simulink model "attitudeEstimation"  (R2018a)
settings: Solver=FixedStepAuto  StartTime=0.0  StopTime=10.0  RelTol=1e-3
undefined symbols (not defined in the file): SkywalkerX8
libraries: sharedTrackingLibrary x1
settings Model: Creator=David  LastModifiedBy=David

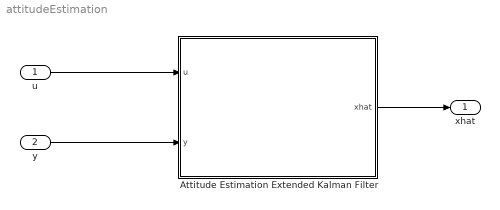
== system attitudeEstimation ==
  u : Inport  PortDimensions=4  SampleTime=SkywalkerX8.Sensors.EKF.Attitude.StateTransitionSampleTime
  y : Inport  Port=2  PortDimensions=3  SampleTime=SkywalkerX8.Sensors.EKF.Attitude.MeasurementSampleTime
  Attitude Estimation Extended Kalman Filter : Subsystem
      mask Display:
      | port_label('input', 1, '{\bf u} = [p, q, r, V_a]', 'texMode', 'On')
      | port_label('input', 2, '{\bf y} = [a_x, a_y, a_z]', 'texMode', 'On')
      | 
      | port_label('output', 1, '{\bf x_{est}} = [\Phi, \theta]', 'texMode', 'On')
  xhat : Outport
  wires:
  u/1 -> Attitude Estimation Extended Kalman Filter/1(u)
  y/1 -> Attitude Estimation Extended Kalman Filter/2(y)
  Attitude Estimation Extended Kalman Filter/1(xhat) -> xhat/1

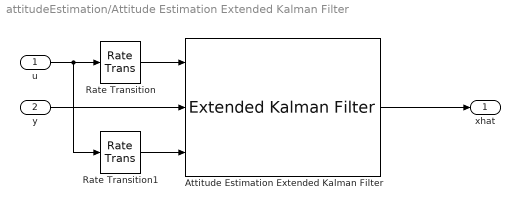
== system attitudeEstimation/Attitude Estimation Extended Kalman Filter ==
  u : Inport
  y : Inport  Port=2
  Attitude Estimation Extended Kalman Filter : sharedTrackingLibrary/Extended Kalman Filter  StateTransitionFcn=attitudeTransitionEstimate  HasStateTransitionJacobianFcn=on  StateTransitionJacobianFcn=attitudeTransitionEstimate_Jacobian  HasAdditiveProcessNoise=Additive  ProcessNoise=SkywalkerX8.Sensors.EKF.Attitude.ProcessCovarianceMatrix  HasTimeVaryingProcessNoise=off  HasStateTransitionFcnExtraArgument=1  InitialState=SkywalkerX8.Sensors.EKF.Attitude.InitialState  InitialStateCovariance=SkywalkerX8.Sensors.EKF.Attitude.InitialStateCovarianceMatrix  MeasurementFcn1=accelerometerMeasurementEstimate  HasMeasurementJacobianFcn1=on  MeasurementJacobianFcn1=accelerometerMeasurementEstimate_Jacobian  HasMeasurementEnablePort1=off  HasAdditiveMeasurementNoise1=Additive  MeasurementNoise1=SkywalkerX8.Sensors.EKF.Attitude.MeasurementCovarianceMatrix  HasTimeVaryingMeasurementNoise1=off  HasMeasurementFcnExtraArgument1=1  MeasurementFcn2=myMeasurementFcn  HasMeasurementJacobianFcn2=off  HasMeasurementEnablePort2=off  HasAdditiveMeasurementNoise2=Additive  MeasurementNoise2=1  HasTimeVaryingMeasurementNoise2=off  HasMeasurementFcnExtraArgument2=0  MeasurementFcn3=myMeasurementFcn  HasMeasurementJacobianFcn3=off  HasMeasurementEnablePort3=off  HasAdditiveMeasurementNoise3=Additive  MeasurementNoise3=1  HasTimeVaryingMeasurementNoise3=off  HasMeasurementFcnExtraArgument3=0  MeasurementFcn4=myMeasurementFcn  HasMeasurementJacobianFcn4=off  HasMeasurementEnablePort4=off  HasAdditiveMeasurementNoise4=Additive  MeasurementNoise4=1  HasTimeVaryingMeasurementNoise4=off  HasMeasurementFcnExtraArgument4=0  MeasurementFcn5=myMeasurementFcn  HasMeasurementJacobianFcn5=off  HasMeasurementEnablePort5=off  HasAdditiveMeasurementNoise5=Additive  MeasurementNoise5=1  HasTimeVaryingMeasurementNoise5=off  HasMeasurementFcnExtraArgument5=0  EnableMultirate=on  StateTransitionFcnSampleTime=SkywalkerX8.Sensors.EKF.Attitude.StateTransitionSampleTime  MeasurementFcn1SampleTime=SkywalkerX8.Sensors.EKF.Attitude.MeasurementSampleTime  MeasurementFcn2SampleTime=1  MeasurementFcn3SampleTime=1  MeasurementFcn4SampleTime=1  MeasurementFcn5SampleTime=1  UseCurrentEstimator=on  OutputStateCovariance=off  DataType=double  SampleTime=SkywalkerX8.Sensors.EKF.Attitude.SampleTime  NumberOfMeasurements=1
      settings: SourceProductName=Control System Toolbox  SourceProductBaseCode=CT
  Rate Transition : RateTransition  OutPortSampleTime=SkywalkerX8.Sensors.EKF.Attitude.StateTransitionSampleTime
  Rate Transition1 : RateTransition  OutPortSampleTime=SkywalkerX8.Sensors.EKF.Attitude.MeasurementSampleTime
  xhat : Outport
  wires:
  y/1 -> Attitude Estimation Extended Kalman Filter/2
  u/1 -> Rate Transition1/1, Rate Transition/1
  Attitude Estimation Extended Kalman Filter/1 -> xhat/1
  Rate Transition/1 -> Attitude Estimation Extended Kalman Filter/1
  Rate Transition1/1 -> Attitude Estimation Extended Kalman Filter/3
